simulink library "lib_transmission2"  (Simulink 10.1)
settings: Solver=VariableStepAuto  StartTime=0.0  StopTime=10.0  RelTol=1e-3
undefined symbols (not defined in the file or in its folder): cyc_mph, fc_map_spd, fc_max_trq, fc_spd_scale, fc_trq_scale, fd_inertia, fd_loss, fd_ratio, gb_gear_number_lookup, gb_gears_num, gb_inertia, gb_loss_const, gb_loss_input_spd_coeff, gb_loss_input_trq_coeff, gb_loss_output_spd_coeff, gb_loss_output_trq_coeff, gb_num_init, gb_ratio, gb_shift_delay, gb_spd_scale, gb_trq_scale, htc_inertia, htc_k_adv, htc_k_adv_coast, htc_lockup, htc_lockup_load, htc_lockup_spd, htc_lu_gear_range, htc_max_coast_tr, htc_min_coast_tr, htc_pump_loss_spd, htc_pump_loss_trq_lockup, htc_pump_loss_trq_unlock, htc_sr, htc_sr_coast, htc_tr, htc_tr_coast, htc_unlock_spd, mc_map_spd, mc_max_trq, mc_overtrq_factor, mc_spd_scale, mc_trq_scale, tc_loss, tc_mc_to_fc_ratio, tx_eff_map, tx_map_spd, tx_map_trq, tx_pg_r, tx_pg_s, tx_speed_dep, vc_clutch_bool, vc_idle_spd, vc_launch_spd, wh_radius
undefined symbols (not defined in the file): gb_dnshift_load, gb_dnshift_spd, gb_map_spd_out, gb_map_trq_in, gb_map_trq_out, gb_upshift_load, gb_upshift_spd, logFlag
libraries: lib_controls x1, lib_etc x1, lib_controls2 x1, lib_transmission x1
(part 12 of 17)

== system lib_transmission2/Gearbox Control/automatic transmission gearbox and htc advanced lock-up logic for htc shift logic for gearbox/gearbox control for use w/ AT/Speed Dependent Shifting ==
  note: storing shifting and gear ratio
      | information to workspace
  note: decel case
  note: accel case
  note: accel
      | case
  note: decel
      | case
  note: delta speed
  note: SPEED
      | DEPENDENT
      | SHIFT
      | SIGNAL
  "velocity required (limited) " : Inport
  Look-Up Table (gear for downshift) : Lookup  InputValues="tx_spd_dep_dnshift(:,1)   % vector of speeds m/s"  Table="tx_spd_dep_dnshift(:,2)  % gear number--must be step function"  SaturateOnIntegerOverflow=on
  Look-Up Table (gear for upshift) : Lookup  InputValues="tx_spd_dep_upshift(:,1)   % vector of speeds in m/s"  Table="tx_spd_dep_upshift(:,2)  % gear number--must be step function"  SaturateOnIntegerOverflow=on
  Mux : Mux  Inputs=2
  Mux2 : Mux  Inputs=2
  New gear ratio : ToWorkspace  VariableName=new_gear_ratio
      settings: MaxDataPoints=50000
  Rounding Function : Rounding  Operator=round
  Rounding Function1 : Rounding  Operator=round
  Saturation4 : Saturate  UpperLimit=gb_gears_num  LowerLimit=1
  Saturation5 : Saturate  UpperLimit=gb_gears_num  LowerLimit=1
  "delta speed (\"+\" is acceleration)" : Sum  Inputs=-+  SaturateOnIntegerOverflow=on
  gear ratio6 : Lookup  InputValues=[1:length(gb_ratio)]  Table=gb_ratio  SaturateOnIntegerOverflow=on
  gear ratio8 : Lookup  InputValues=[1:length(gb_ratio)]  Table=gb_ratio  SaturateOnIntegerOverflow=on
  prev veh speed : Memory  InitialCondition=1
  shifting : Subsystem  AncestorBlock=lib_controls/SubSystem/shifting
  shifting1 : Subsystem  AncestorBlock=lib_controls/SubSystem/shifting
  switch for gear number : Switch  Threshold=eps  SaturateOnIntegerOverflow=on  InputSameDT=on
  switch for gear ratio and shifting (muxed) : Switch  Threshold=eps  SaturateOnIntegerOverflow=on  InputSameDT=on
  total fuel used (gal) : ToWorkspace  VariableName=neg_gear_num
      settings: MaxDataPoints=50000
  gear ratio and shifting : Outport
  gear number : Outport  Port=2
  wires:
  Rounding Function1/1 -> Saturation5/1
  Look-Up Table (gear for downshift)/1 -> Rounding Function1/1
  Rounding Function/1 -> Saturation4/1
  Look-Up Table (gear for upshift)/1 -> Rounding Function/1
  "delta speed (\"+\" is acceleration)"/1 -> switch for gear ratio and shifting (muxed)/2, switch for gear number/2
  switch for gear number/1 -> gear number/1
  switch for gear ratio and shifting (muxed)/1 -> gear ratio and shifting/1, New gear ratio/1
  Saturation4/1 -> gear ratio6/1, shifting1/1(gear number), switch for gear number/1
  shifting1/1(out_1) -> Mux/2
  gear ratio6/1 -> Mux/1
  Saturation5/1 -> shifting/1(gear number), gear ratio8/1, total fuel used (gal)/1, switch for gear number/3
  gear ratio8/1 -> Mux2/1
  shifting/1(out_1) -> Mux2/2
  Mux/1 -> switch for gear ratio and shifting (muxed)/1
  Mux2/1 -> switch for gear ratio and shifting (muxed)/3
  prev veh speed/1 -> "delta speed (\"+\" is acceleration)"/1
  "velocity required (limited) "/1 -> Look-Up Table (gear for upshift)/1, Look-Up Table (gear for downshift)/1, "delta speed (\"+\" is acceleration)"/2, prev veh speed/1

== system lib_transmission2/Gearbox Control/automatic transmission gearbox and htc advanced lock-up logic for htc shift logic for gearbox/gearbox control for use w/ AT/allow downshift? ==
  prev gearnum : Inport
  Logical Operator : Logic  Operator=NOR
  Memory : Memory  InitialCondition=1
  Memory1 : Memory  InitialCondition=1
  Relational Operator1 : RelationalOperator  Operator=>  RndMeth=Nearest  InputSameDT=on
  Relational Operator2 : RelationalOperator  Operator=>  RndMeth=Nearest  InputSameDT=on
  allow shift : Outport  InitialOutput=0
  wires:
  Logical Operator/1 -> allow shift/1
  prev gearnum/1 -> Relational Operator1/1, Memory/1, Relational Operator2/1
  Relational Operator1/1 -> Logical Operator/1
  Memory/1 -> Relational Operator1/2, Memory1/1
  Memory1/1 -> Relational Operator2/2
  Relational Operator2/1 -> Logical Operator/2

== system lib_transmission2/Gearbox Control/automatic transmission gearbox and htc advanced lock-up logic for htc shift logic for gearbox/gearbox control for use w/ AT/downshift  command ==
  prev gear number : Inport
  engine load : Inport  Port=2
  engine speed : Inport  Port=3
  Mux : Mux  Inputs=2
  Relational Operator : RelationalOperator  Operator=>  RndMeth=Nearest  InputSameDT=on
  load fraction : Subsystem  mask(Gear Selector){spd=gb_dnshift_spd, load=gb_dnshift_load}
      mask prompts: spd "Speeds:"; load "Load Fractions:"
      mask help:
      | This block will perform a linear interplation (extrapolation outside of bounds) to determine the shift point load fraction associated with the current gear number and speed.
      |
      | The Speeds parameter should be defined as an array of vectors containing speeds for each gear number.  The Load Fractions parameter should be defined as a array of vectors containing load fractions indexed by the speeds in the Speeds parameter for each gear number.
      mask Help:
      | Reference the base workspace variables - gb_**shift_spd and gb_**shift_load  where ** is either up for upshift conditions or dn for downshift conditions.
      | 
      | Or define the arrays as follows:
      | 
      | {[spd1 spd2 spd3 spd4]; [spd1 spd2 spd3 spd4]; ...}
      | 
      | {[load1 load2 load3 load4]; [load1 load2 load3 load4]; ...}
      | 
      | where each array contains one row for each gear in the gearbox.  Speeds should be defined in rad/s and loads as a decimal fraction.
  command : Outport  InitialOutput=0
  wires:
  Relational Operator/1 -> command/1
  engine speed/1 -> Mux/2
  prev gear number/1 -> Mux/1
  engine load/1 -> Relational Operator/1
  Mux/1 -> load fraction/1(In1)
  load fraction/1(Out1) -> Relational Operator/2

== system lib_transmission2/Gearbox Control/automatic transmission gearbox and htc advanced lock-up logic for htc shift logic for gearbox/gearbox control for use w/ AT/downshift  command1 ==
  prev gear number : Inport
  engine load : Inport  Port=2
  engine speed : Inport  Port=3
  Mux : Mux  Inputs=2
  Relational Operator : RelationalOperator  Operator=>  RndMeth=Nearest  InputSameDT=on
  load fraction : Subsystem  mask(Gear Selector){spd=gb_dnshift_spd, load=gb_dnshift_load}
      mask prompts: spd "Speeds:"; load "Load Fractions:"
      mask help:
      | This block will perform a linear interplation (extrapolation outside of bounds) to determine the shift point load fraction associated with the current gear number and speed.
      |
      | The Speeds parameter should be defined as an array of vectors containing speeds for each gear number.  The Load Fractions parameter should be defined as a array of vectors containing load fractions indexed by the speeds in the Speeds parameter for each gear number.
      mask Help:
      | Reference the base workspace variables - gb_**shift_spd and gb_**shift_load  where ** is either up for upshift conditions or dn for downshift conditions.
      | 
      | Or define the arrays as follows:
      | 
      | {[spd1 spd2 spd3 spd4]; [spd1 spd2 spd3 spd4]; ...}
      | 
      | {[load1 load2 load3 load4]; [load1 load2 load3 load4]; ...}
      | 
      | where each array contains one row for each gear in the gearbox.  Speeds should be defined in rad/s and loads as a decimal fraction.
  command : Outport  InitialOutput=0
  wires:
  engine speed/1 -> Mux/2
  load fraction/1(Out1) -> Relational Operator/2
  Mux/1 -> load fraction/1(In1)
  engine load/1 -> Relational Operator/1
  prev gear number/1 -> Mux/1
  Relational Operator/1 -> command/1

== system lib_transmission2/Gearbox Control/automatic transmission gearbox and htc advanced lock-up logic for htc shift logic for gearbox/gearbox control for use w/ AT/est. engine trq and spd ==
  prev gear number : Inport
  " prev eta_gb" : Inport  Port=2
  gb_trq_out_r : Inport  Port=3
  gb_spd_out_r : Inport  Port=4
  Block NOTES : Subsystem
      mask Display: disp('Block\nNOTES')
  Constant2 : Constant  Value=[1 1]
  Constant5 : Constant  Value=0
  Demux : Demux  Outputs=2
  K_adv : Subsystem
  Logical Operator : Logic
  Logical Operator1 : Logic  Operator=NOT  Inputs=1
  Memory : Memory
  Mux1 : Mux  Inputs=2
  Mux2 : Mux  Inputs=2
  Relational Operator1 : RelationalOperator  Operator=>  RndMeth=Nearest  InputSameDT=on
  SR Look-Up Table SR=wout/win : Lookup  InputValues=htc_k_adv  Table=htc_sr  SaturateOnIntegerOverflow=on
  Saturation1 : Saturate  UpperLimit=1  LowerLimit=0.7
  Saturation2 : Saturate  UpperLimit=inf  LowerLimit=0
  Switch : Switch  Threshold=eps  SaturateOnIntegerOverflow=on  InputSameDT=on
  TR Look-Up Table TR=Tout/Tin : Lookup  InputValues=htc_k_adv  Table=htc_tr  SaturateOnIntegerOverflow=on
  TR,SR : Mux  Inputs=2
  est eng trq : Sum  SaturateOnIntegerOverflow=on
  gear ratio1 : Lookup  InputValues=[1:length(gb_ratio)]  Table=gb_ratio  SaturateOnIntegerOverflow=on
  ~eng trq and spd : Product  Inputs=*/  SaturateOnIntegerOverflow=on
  ~gb_spd_in_r : Product  SaturateOnIntegerOverflow=on
  ~gb_trq_in_r : Product  Inputs=//*  SaturateOnIntegerOverflow=on
  est eng trq (Nm) : Outport
  est eng spd (rad/s) : Outport  Port=2
  gb_spd_in_est (rad/s)1 : Outport  Port=3
  wires:
  est eng trq/1 -> Mux1/1, Relational Operator1/1, Mux2/1
  ~gb_trq_in_r/1 -> est eng trq/1
  ~gb_spd_in_r/1 -> Mux2/2, gb_spd_in_est (rad/s)1/1, Mux1/2
  [acc_mech_trq_est] -> est eng trq/2
  SR Look-Up Table SR=wout/win/1 -> TR,SR/2
  TR Look-Up Table TR=Tout/Tin/1 -> TR,SR/1
  K_adv/1(K_adv) -> SR Look-Up Table SR=wout/win/1, TR Look-Up Table TR=Tout/Tin/1
  Mux2/1 -> K_adv/1("Req'd output trq and spd (Nm), (rad/s)")
  ~eng trq and spd/1 -> Demux/1
  Mux1/1 -> ~eng trq and spd/1
  [locked_up] -> Memory/1
  Logical Operator/1 -> Switch/2
  Logical Operator1/1 -> Logical Operator/2
  Memory/1 -> Logical Operator1/1
  Demux/1 -> est eng trq (Nm)/1
  prev gear number/1 -> gear ratio1/1
  Relational Operator1/1 -> Logical Operator/1
  Constant5/1 -> Relational Operator1/2
  Saturation2/1 -> est eng spd (rad/s)/1
  Demux/2 -> Saturation2/1
  Saturation1/1 -> ~gb_trq_in_r/2
  " prev eta_gb"/1 -> Saturation1/1
  Switch/1 -> ~eng trq and spd/2
  Constant2/1 -> Switch/3
  TR,SR/1 -> Switch/1
  gear ratio1/1 -> ~gb_spd_in_r/1, ~gb_trq_in_r/1
  gb_spd_out_r/1 -> ~gb_spd_in_r/2
  gb_trq_out_r/1 -> ~gb_trq_in_r/3

== system lib_transmission2/Gearbox Control/automatic transmission gearbox and htc advanced lock-up logic for htc shift logic for gearbox/gearbox control for use w/ AT/est. engine trq and spd assuming lockup ==
  new gear number : Inport
  " prev eta_gb" : Inport  Port=2
  gb_trq_out_r : Inport  Port=3
  gb_spd_in_est : Inport  Port=4
  Block NOTES : Subsystem
      mask Display: disp('Block\nNOTES')
  Memory : Memory  InitialCondition=gb_ratio(1)
  Saturation1 : Saturate  UpperLimit=1  LowerLimit=0.7
  Saturation2 : Saturate  UpperLimit=inf  LowerLimit=0
  est eng trq : Sum  SaturateOnIntegerOverflow=on
  gear ratio1 : Lookup  InputValues=[1:length(gb_ratio)]  Table=gb_ratio  SaturateOnIntegerOverflow=on
  ~gb_spd_in_r : Product  Inputs=*/*  SaturateOnIntegerOverflow=on
  ~gb_trq_in_r : Product  Inputs=//*  SaturateOnIntegerOverflow=on
  est eng trq (Nm) : Outport
  est eng spd (rad/s) : Outport  Port=2
  wires:
  ~gb_spd_in_r/1 -> Saturation2/1
  est eng trq/1 -> est eng trq (Nm)/1
  ~gb_trq_in_r/1 -> est eng trq/1
  [acc_mech_trq_est] -> est eng trq/2
  gb_spd_in_est/1 -> ~gb_spd_in_r/3
  Memory/1 -> ~gb_spd_in_r/2
  Saturation2/1 -> est eng spd (rad/s)/1
  new gear number/1 -> gear ratio1/1
  gb_trq_out_r/1 -> ~gb_trq_in_r/3
  gear ratio1/1 -> Memory/1, ~gb_spd_in_r/1, ~gb_trq_in_r/1
  " prev eta_gb"/1 -> Saturation1/1
  Saturation1/1 -> ~gb_trq_in_r/2

== system lib_transmission2/Gearbox Control/automatic transmission gearbox and htc advanced lock-up logic for htc shift logic for gearbox/gearbox control for use w/ AT/htc lockup logic ==
  engine load (%) : Inport
  gear num : Inport  Port=2
  Constant1 : Constant  Value=0.5
  Constant2 : Constant  Value=0
  Constant3 : Constant  Value=0
  Constant4 : Constant  Value=-1
  Logical Operator : Logic  Operator=NOR
  Memory1 : Memory  InitialCondition=1
  Memory2 : Memory  InitialCondition=1
  Memory3 : Memory  InitialCondition=1
  Relational Operator : RelationalOperator  RndMeth=Nearest  InputSameDT=on
  Relational Operator1 : RelationalOperator  Operator=>  RndMeth=Nearest  InputSameDT=on
  Relational Operator2 : RelationalOperator  Operator=<  RndMeth=Nearest  InputSameDT=on
  Relational Operator3 : RelationalOperator  Operator=<  RndMeth=Nearest  InputSameDT=on
  Saturation1 : Saturate  UpperLimit=1  LowerLimit=0
  Switch{,1..3} (4 alike) : Switch  Threshold=0.5  SaturateOnIntegerOverflow=on  InputSameDT=on
  current lock/unlock  status : Sum  SaturateOnIntegerOverflow=on
  lock-up in high gears : Lookup  InputValues=[1:length(htc_lockup)]  Table=htc_lockup  SaturateOnIntegerOverflow=on
  lock-up in this gear : Lookup  InputValues=htc_lockup_load  Table=htc_lockup_spd  SaturateOnIntegerOverflow=on
  lock/unlock  gear range : Lookup  InputValues=[1:length(htc_lockup)]  Table=htc_lu_gear_range  SaturateOnIntegerOverflow=on
  unlock in this gear : Lookup  InputValues=htc_lockup_load  Table=htc_unlock_spd  SaturateOnIntegerOverflow=on
  htc L/UL : Outport
  wires:
  Constant1/1 -> Relational Operator/2, Relational Operator1/1
  gear num/1 -> lock-up in high gears/1, lock/unlock  gear range/1
  lock-up in high gears/1 -> Relational Operator/1
  Relational Operator/1 -> Switch/2, Switch/1
  Switch/1 -> htc L/UL/1, Memory1/1
  lock/unlock  gear range/1 -> Relational Operator1/2
  lock-up in this gear/1 -> Relational Operator2/1
  unlock in this gear/1 -> Relational Operator3/2
  Relational Operator1/1 -> Switch1/2
  Constant2/1 -> Switch1/1
  Switch1/1 -> Switch/3
  Saturation1/1 -> Switch1/3
  Relational Operator2/1 -> Logical Operator/1, Switch3/2, Switch3/1
  Relational Operator3/1 -> Logical Operator/2
  Logical Operator/1 -> Switch2/2
  Constant3/1 -> Switch2/3
  Switch3/1 -> Switch2/1
  Constant4/1 -> Switch3/3
  current lock/unlock  status/1 -> Saturation1/1
  Memory1/1 -> current lock/unlock  status/1
  Switch2/1 -> current lock/unlock  status/2
  Memory2/1 -> Relational Operator2/2, Relational Operator3/1
  Memory3/1 -> lock-up in this gear/1, unlock in this gear/1
  engine load (%)/1 -> Memory3/1
  [gb_trq_out_a] -> Memory2/1

== system lib_transmission2/Gearbox Control/automatic transmission gearbox and htc advanced lock-up logic for htc shift logic for gearbox/gearbox control for use w/ AT/shifting1 ==
  gear number : Inport
  Constant : Constant  Value=gb_shift_delay-1e-6
  Relational Operator : RelationalOperator  Operator=<  RndMeth=Nearest  InputSameDT=on
  time since last shift : Subsystem
      mask Display: disp('time since\nlast shift')
  out_1 : Outport  InitialOutput=0
  wires:
  Relational Operator/1 -> out_1/1
  gear number/1 -> time since last shift/1(in_1)
  Constant/1 -> Relational Operator/2
  time since last shift/1(out_1) -> Relational Operator/1

== system lib_transmission2/Gearbox Control/automatic transmission gearbox and htc advanced lock-up logic for htc shift logic for gearbox/gearbox control for use w/ AT/upshift  command ==
  prev gear number : Inport
  engine load : Inport  Port=2
  engine speed : Inport  Port=3
  Mux : Mux  Inputs=2
  Relational Operator : RelationalOperator  Operator=<  RndMeth=Nearest  InputSameDT=on
  load fraction : Subsystem  mask(Gear Selector){spd=gb_upshift_spd, load=gb_upshift_load}
      mask prompts: spd "Speeds:"; load "Load Fractions:"
      mask help:
      | This block will perform a linear interplation (extrapolation outside of bounds) to determine the shift point load fraction associated with the current gear number and speed.
      |
      | The Speeds parameter should be defined as an array of vectors containing speeds for each gear number.  The Load Fractions parameter should be defined as a array of vectors containing load fractions indexed by the speeds in the Speeds parameter for each gear number.
      mask Help:
      | Reference the base workspace variables - gb_**shift_spd and gb_**shift_load  where ** is either up for upshift conditions or dn for downshift conditions.
      | 
      | Or define the arrays as follows:
      | 
      | {[spd1 spd2 spd3 spd4]; [spd1 spd2 spd3 spd4]; ...}
      | 
      | {[load1 load2 load3 load4]; [load1 load2 load3 load4]; ...}
      | 
      | where each array contains one row for each gear in the gearbox.  Speeds should be defined in rad/s and loads as a decimal fraction.
  command : Outport  InitialOutput=0
  wires:
  Relational Operator/1 -> command/1
  engine speed/1 -> Mux/2
  Mux/1 -> load fraction/1(In1)
  prev gear number/1 -> Mux/1
  engine load/1 -> Relational Operator/1
  load fraction/1(Out1) -> Relational Operator/2

== system lib_transmission2/Gearbox Control/automatic transmission gearbox and htc standard lockup logic for htc shift logic for gearbox/gearbox control for use w/ AT/Block NOTES ==
  note: This gearbox control block computes the current gear number given the gearbox's
      | req'd output torque and speed and an estimate its efficiency.  Upshifts occur, given a
      | certain engine speed,  when the estimated engine load falls below the upshift curve
      | in engine speed/load space, and downshifts likewise occur when estimated engine
      | load rises above the downshift curve.  Separate upshift and downshift curves are
      | defined for each gear.  An upshift may not be immediately followed by a downshift.
      | If the tires are about to slip, don't upshift unless the engine would be at max. speed.
      | Enforce this rule by setting the load to 1 when the tires are about to slip.
  note: Lock-up of the HTC occurs when it is supposed to for the current gear, AND
      | the transmission isn't shifting, AND
      | the lockup wouldn't precipitate an immediate downshift.

== system lib_transmission2/Gearbox Control/automatic transmission gearbox and htc standard lockup logic for htc shift logic for gearbox/gearbox control for use w/ AT/allow downshift? ==
  prev gearnum : Inport
  Logical Operator : Logic  Operator=NOR
  Memory : Memory  InitialCondition=1
  Memory1 : Memory  InitialCondition=1
  Relational Operator1 : RelationalOperator  Operator=>  RndMeth=Nearest  InputSameDT=on
  Relational Operator2 : RelationalOperator  Operator=>  RndMeth=Nearest  InputSameDT=on
  allow shift : Outport  InitialOutput=0
  wires:
  Relational Operator2/1 -> Logical Operator/2
  Memory1/1 -> Relational Operator2/2
  Memory/1 -> Memory1/1, Relational Operator1/2
  Relational Operator1/1 -> Logical Operator/1
  prev gearnum/1 -> Relational Operator2/1, Memory/1, Relational Operator1/1
  Logical Operator/1 -> allow shift/1

== system lib_transmission2/Gearbox Control/automatic transmission gearbox and htc standard lockup logic for htc shift logic for gearbox/gearbox control for use w/ AT/downshift  command ==
  prev gear number : Inport
  engine load : Inport  Port=2
  engine speed : Inport  Port=3
  Mux : Mux  Inputs=2
  Relational Operator : RelationalOperator  Operator=>  RndMeth=Nearest  InputSameDT=on
  load fraction : Subsystem  mask(Gear Selector){spd=gb_dnshift_spd, load=gb_dnshift_load}
      mask prompts: spd "Speeds:"; load "Load Fractions:"
      mask help:
      | This block will perform a linear interplation (extrapolation outside of bounds) to determine the shift point load fraction associated with the current gear number and speed.
      |
      | The Speeds parameter should be defined as an array of vectors containing speeds for each gear number.  The Load Fractions parameter should be defined as a array of vectors containing load fractions indexed by the speeds in the Speeds parameter for each gear number.
      mask Help:
      | Reference the base workspace variables - gb_**shift_spd and gb_**shift_load  where ** is either up for upshift conditions or dn for downshift conditions.
      | 
      | Or define the arrays as follows:
      | 
      | {[spd1 spd2 spd3 spd4]; [spd1 spd2 spd3 spd4]; ...}
      | 
      | {[load1 load2 load3 load4]; [load1 load2 load3 load4]; ...}
      | 
      | where each array contains one row for each gear in the gearbox.  Speeds should be defined in rad/s and loads as a decimal fraction.
  command : Outport  InitialOutput=0
  wires:
  load fraction/1(Out1) -> Relational Operator/2
  Mux/1 -> load fraction/1(In1)
  engine load/1 -> Relational Operator/1
  prev gear number/1 -> Mux/1
  engine speed/1 -> Mux/2
  Relational Operator/1 -> command/1

== system lib_transmission2/Gearbox Control/automatic transmission gearbox and htc standard lockup logic for htc shift logic for gearbox/gearbox control for use w/ AT/downshift  command1 ==
  prev gear number : Inport
  engine load : Inport  Port=2
  engine speed : Inport  Port=3
  Mux : Mux  Inputs=2
  Relational Operator : RelationalOperator  Operator=>  RndMeth=Nearest  InputSameDT=on
  load fraction : Subsystem  mask(Gear Selector){spd=gb_dnshift_spd, load=gb_dnshift_load}
      mask prompts: spd "Speeds:"; load "Load Fractions:"
      mask help:
      | This block will perform a linear interplation (extrapolation outside of bounds) to determine the shift point load fraction associated with the current gear number and speed.
      |
      | The Speeds parameter should be defined as an array of vectors containing speeds for each gear number.  The Load Fractions parameter should be defined as a array of vectors containing load fractions indexed by the speeds in the Speeds parameter for each gear number.
      mask Help:
      | Reference the base workspace variables - gb_**shift_spd and gb_**shift_load  where ** is either up for upshift conditions or dn for downshift conditions.
      | 
      | Or define the arrays as follows:
      | 
      | {[spd1 spd2 spd3 spd4]; [spd1 spd2 spd3 spd4]; ...}
      | 
      | {[load1 load2 load3 load4]; [load1 load2 load3 load4]; ...}
      | 
      | where each array contains one row for each gear in the gearbox.  Speeds should be defined in rad/s and loads as a decimal fraction.
  command : Outport  InitialOutput=0
  wires:
  Relational Operator/1 -> command/1
  prev gear number/1 -> Mux/1
  engine load/1 -> Relational Operator/1
  Mux/1 -> load fraction/1(In1)
  load fraction/1(Out1) -> Relational Operator/2
  engine speed/1 -> Mux/2

== system lib_transmission2/Gearbox Control/automatic transmission gearbox and htc standard lockup logic for htc shift logic for gearbox/gearbox control for use w/ AT/est. engine trq and spd ==
  prev gear number : Inport
  " prev eta_gb" : Inport  Port=2
  gb_trq_out_r : Inport  Port=3
  gb_spd_out_r : Inport  Port=4
  Block NOTES : Subsystem
      mask Display: disp('Block\nNOTES')
  Constant2 : Constant  Value=[1 1]
  Constant5 : Constant  Value=0
  Demux : Demux  Outputs=2
  K_adv : Subsystem
  Logical Operator : Logic
  Logical Operator1 : Logic  Operator=NOT  Inputs=1
  Mux1 : Mux  Inputs=2
  Mux2 : Mux  Inputs=2
  Relational Operator1 : RelationalOperator  Operator=>  RndMeth=Nearest  InputSameDT=on
  SR Look-Up Table SR=wout/win : Lookup  InputValues=htc_k_adv  Table=htc_sr  SaturateOnIntegerOverflow=on
  Saturation1 : Saturate  UpperLimit=1  LowerLimit=0.7
  Saturation2 : Saturate  UpperLimit=inf  LowerLimit=0
  Switch : Switch  Threshold=eps  SaturateOnIntegerOverflow=on  InputSameDT=on
  TR Look-Up Table TR=Tout/Tin : Lookup  InputValues=htc_k_adv  Table=htc_tr  SaturateOnIntegerOverflow=on
  TR,SR : Mux  Inputs=2
  est eng trq : Sum  SaturateOnIntegerOverflow=on
  gear ratio : Lookup  InputValues=[1:length(gb_ratio)]  Table=gb_ratio  SaturateOnIntegerOverflow=on
  ~eng trq and spd : Product  Inputs=*/  SaturateOnIntegerOverflow=on
  ~gb_spd_in_r : Product  SaturateOnIntegerOverflow=on
  ~gb_trq_in_r : Product  Inputs=//*  SaturateOnIntegerOverflow=on
  est eng trq (Nm) : Outport
  est eng spd (rad/s) : Outport  Port=2
  gb_spd_in_est (rad/s) : Outport  Port=3
  wires:
  gb_trq_out_r/1 -> ~gb_trq_in_r/3
  gb_spd_out_r/1 -> ~gb_spd_in_r/2
  gear ratio/1 -> ~gb_trq_in_r/1, ~gb_spd_in_r/1
  TR,SR/1 -> Switch/1
  Constant2/1 -> Switch/3
  Switch/1 -> ~eng trq and spd/2
  " prev eta_gb"/1 -> Saturation1/1
  Saturation1/1 -> ~gb_trq_in_r/2
  Demux/2 -> Saturation2/1
  Saturation2/1 -> est eng spd (rad/s)/1
  Constant5/1 -> Relational Operator1/2
  Relational Operator1/1 -> Logical Operator/1
  prev gear number/1 -> gear ratio/1
  Demux/1 -> est eng trq (Nm)/1
  Logical Operator1/1 -> Logical Operator/2
  Logical Operator/1 -> Switch/2
  [locked_up_last] -> Logical Operator1/1
  Mux1/1 -> ~eng trq and spd/1
  ~eng trq and spd/1 -> Demux/1
  Mux2/1 -> K_adv/1("Req'd output trq and spd (Nm), (rad/s)")
  K_adv/1(K_adv) -> TR Look-Up Table TR=Tout/Tin/1, SR Look-Up Table SR=wout/win/1
  TR Look-Up Table TR=Tout/Tin/1 -> TR,SR/1
  SR Look-Up Table SR=wout/win/1 -> TR,SR/2
  [acc_mech_trq_est] -> est eng trq/2
  ~gb_spd_in_r/1 -> Mux1/2, gb_spd_in_est (rad/s)/1, Mux2/2
  ~gb_trq_in_r/1 -> est eng trq/1
  est eng trq/1 -> Mux2/1, Relational Operator1/1, Mux1/1

== system lib_transmission2/Gearbox Control/automatic transmission gearbox and htc standard lockup logic for htc shift logic for gearbox/gearbox control for use w/ AT/est. engine trq and spd assuming lockup ==
  new gear number : Inport
  " prev eta_gb" : Inport  Port=2
  gb_trq_out_r : Inport  Port=3
  gb_spd_in_est : Inport  Port=4
  Block NOTES : Subsystem
      mask Display: disp('Block\nNOTES')
  Memory : Memory  InitialCondition=gb_ratio(1)
  Saturation1 : Saturate  UpperLimit=1  LowerLimit=0.7
  Saturation2 : Saturate  UpperLimit=inf  LowerLimit=0
  est eng trq : Sum  SaturateOnIntegerOverflow=on
  gear ratio1 : Lookup  InputValues=[1:length(gb_ratio)]  Table=gb_ratio  SaturateOnIntegerOverflow=on
  ~gb_spd_in_r : Product  Inputs=*/*  SaturateOnIntegerOverflow=on
  ~gb_trq_in_r : Product  Inputs=//*  SaturateOnIntegerOverflow=on
  est eng trq (Nm) : Outport
  est eng spd (rad/s) : Outport  Port=2
  wires:
  Saturation1/1 -> ~gb_trq_in_r/2
  " prev eta_gb"/1 -> Saturation1/1
  gear ratio1/1 -> ~gb_trq_in_r/1, ~gb_spd_in_r/1, Memory/1
  gb_trq_out_r/1 -> ~gb_trq_in_r/3
  new gear number/1 -> gear ratio1/1
  Saturation2/1 -> est eng spd (rad/s)/1
  Memory/1 -> ~gb_spd_in_r/2
  gb_spd_in_est/1 -> ~gb_spd_in_r/3
  [acc_mech_trq_est] -> est eng trq/2
  ~gb_trq_in_r/1 -> est eng trq/1
  est eng trq/1 -> est eng trq (Nm)/1
  ~gb_spd_in_r/1 -> Saturation2/1

== system lib_transmission2/Gearbox Control/automatic transmission gearbox and htc standard lockup logic for htc shift logic for gearbox/gearbox control for use w/ AT/shifting1 ==
  gear number : Inport
  Constant : Constant  Value=gb_shift_delay-1e-6
  Relational Operator : RelationalOperator  Operator=<  RndMeth=Nearest  InputSameDT=on
  time since last shift : Subsystem
      mask Display: disp('time since\nlast shift')
  out_1 : Outport  InitialOutput=0
  wires:
  time since last shift/1(out_1) -> Relational Operator/1
  Constant/1 -> Relational Operator/2
  gear number/1 -> time since last shift/1(in_1)
  Relational Operator/1 -> out_1/1

== system lib_transmission2/Gearbox Control/automatic transmission gearbox and htc standard lockup logic for htc shift logic for gearbox/gearbox control for use w/ AT/upshift  command ==
  prev gear number : Inport
  engine load : Inport  Port=2
  engine speed : Inport  Port=3
  Mux : Mux  Inputs=2
  Relational Operator : RelationalOperator  Operator=<  RndMeth=Nearest  InputSameDT=on
  load fraction : Subsystem  mask(Gear Selector){spd=gb_upshift_spd, load=gb_upshift_load}
      mask prompts: spd "Speeds:"; load "Load Fractions:"
      mask help:
      | This block will perform a linear interplation (extrapolation outside of bounds) to determine the shift point load fraction associated with the current gear number and speed.
      |
      | The Speeds parameter should be defined as an array of vectors containing speeds for each gear number.  The Load Fractions parameter should be defined as a array of vectors containing load fractions indexed by the speeds in the Speeds parameter for each gear number.
      mask Help:
      | Reference the base workspace variables - gb_**shift_spd and gb_**shift_load  where ** is either up for upshift conditions or dn for downshift conditions.
      | 
      | Or define the arrays as follows:
      | 
      | {[spd1 spd2 spd3 spd4]; [spd1 spd2 spd3 spd4]; ...}
      | 
      | {[load1 load2 load3 load4]; [load1 load2 load3 load4]; ...}
      | 
      | where each array contains one row for each gear in the gearbox.  Speeds should be defined in rad/s and loads as a decimal fraction.
  command : Outport  InitialOutput=0
  wires:
  load fraction/1(Out1) -> Relational Operator/2
  engine load/1 -> Relational Operator/1
  prev gear number/1 -> Mux/1
  Mux/1 -> load fraction/1(In1)
  engine speed/1 -> Mux/2
  Relational Operator/1 -> command/1

== system lib_transmission2/Gearbox Control/time lookup shift logic for gearbox/lookup/shifting determination ==
  gear number : Inport
  Constant : Constant  Value=gb_shift_delay-1e-6
  Relational Operator : RelationalOperator  Operator=<  RndMeth=Nearest  InputSameDT=on
  time since last shift : Subsystem
      mask Display: disp('time since\nlast shift')
  out_1 : Outport  InitialOutput=0
  wires:
  time since last shift/1(out_1) -> Relational Operator/1
  Constant/1 -> Relational Operator/2
  gear number/1 -> time since last shift/1(in_1)
  Relational Operator/1 -> out_1/1

== system lib_transmission2/Gearbox Control/vehicle speed dependent shift logic for gearbox/speed dependent/Speed Dependent Shifting ==
  note: storing shifting and gear ratio
      | information to workspace
  note: decel case
  note: accel case
  note: accel
      | case
  note: decel
      | case
  note: delta speed
  note: SPEED
      | DEPENDENT
      | SHIFT
      | SIGNAL
  "velocity required (limited) " : Inport
  Look-Up Table (gear for downshift) : Lookup  InputValues="tx_spd_dep_dnshift(:,1)   % vector of speeds m/s"  Table="tx_spd_dep_dnshift(:,2)  % gear number--must be step function"  SaturateOnIntegerOverflow=on
  Look-Up Table (gear for upshift) : Lookup  InputValues="tx_spd_dep_upshift(:,1)   % vector of speeds in m/s"  Table="tx_spd_dep_upshift(:,2)  % gear number--must be step function"  SaturateOnIntegerOverflow=on
  Mux : Mux  Inputs=2
  Mux2 : Mux  Inputs=2
  New gear ratio : ToWorkspace  VariableName=new_gear_ratio
      settings: MaxDataPoints=50000
  Rounding Function : Rounding  Operator=round
  Rounding Function1 : Rounding  Operator=round
  Saturation4 : Saturate  UpperLimit=gb_gears_num  LowerLimit=1
  Saturation5 : Saturate  UpperLimit=gb_gears_num  LowerLimit=1
  "delta speed (\"+\" is acceleration)" : Sum  Inputs=-+  SaturateOnIntegerOverflow=on
  gear ratio6 : Lookup  InputValues=[1:length(gb_ratio)]  Table=gb_ratio  SaturateOnIntegerOverflow=on
  gear ratio8 : Lookup  InputValues=[1:length(gb_ratio)]  Table=gb_ratio  SaturateOnIntegerOverflow=on
  prev veh speed : Memory  InitialCondition=1
  shifting : Subsystem
  shifting1 : Subsystem
  switch for gear number : Switch  Threshold=eps  SaturateOnIntegerOverflow=on  InputSameDT=on
  switch for gear ratio and shifting (muxed) : Switch  Threshold=eps  SaturateOnIntegerOverflow=on  InputSameDT=on
  total fuel used (gal) : ToWorkspace  VariableName=neg_gear_num
      settings: MaxDataPoints=50000
  gear ratio and shifting : Outport
  gear number : Outport  Port=2
  wires:
  Rounding Function1/1 -> Saturation5/1
  Look-Up Table (gear for downshift)/1 -> Rounding Function1/1
  Rounding Function/1 -> Saturation4/1
  Look-Up Table (gear for upshift)/1 -> Rounding Function/1
  "delta speed (\"+\" is acceleration)"/1 -> switch for gear ratio and shifting (muxed)/2, switch for gear number/2
  switch for gear number/1 -> gear number/1
  switch for gear ratio and shifting (muxed)/1 -> gear ratio and shifting/1, New gear ratio/1
  Saturation4/1 -> gear ratio6/1, shifting1/1(gear number), switch for gear number/1
  shifting1/1(out_1) -> Mux/2
  gear ratio6/1 -> Mux/1
  Saturation5/1 -> shifting/1(gear number), gear ratio8/1, total fuel used (gal)/1, switch for gear number/3
  gear ratio8/1 -> Mux2/1
  shifting/1(out_1) -> Mux2/2
  Mux/1 -> switch for gear ratio and shifting (muxed)/1
  Mux2/1 -> switch for gear ratio and shifting (muxed)/3
  prev veh speed/1 -> "delta speed (\"+\" is acceleration)"/1
  "velocity required (limited) "/1 -> Look-Up Table (gear for upshift)/1, Look-Up Table (gear for downshift)/1, "delta speed (\"+\" is acceleration)"/2, prev veh speed/1

== system lib_transmission2/clutch <cl>/clutch model and interface/clutch model/Adjust for Possible Launch Speed Request ==
  note: If the clutch is disengaged, under certain
      | circumstances, we will want to request that
      | the input speed to the clutch be ramped up to a
      | given launch speed (decided by the controller)
      | so that the clutch can subsequently slip and
      | engage with a more realistic speed matching
  Input Speed Request : Inport
  Constant6 : Constant
  Logical Operator : Logic
  Switch4 : Switch  Threshold=0.5  SaturateOnIntegerOverflow=on  InputSameDT=on
  clutch disengaged : RelationalOperator  Operator===  RndMeth=Nearest  InputSameDT=on
  Input Speed Request Adjusted for Launch Speed : Outport
  wires:
  [launch_speed] -> Switch4/1
  Switch4/1 -> Input Speed Request Adjusted for Launch Speed/1
  Input Speed Request/1 -> Switch4/3
  [clutch_state] -> clutch disengaged/1
  Constant6/1 -> clutch disengaged/2
  [launch_flag] -> Logical Operator/1
  clutch disengaged/1 -> Logical Operator/2
  Logical Operator/1 -> Switch4/2

== system lib_transmission2/clutch <cl>/clutch model and interface/clutch model/enhancedToWorkspace ==
  In1 : Inport
  Terminator : Terminator
  wires:
  In1/1 -> Terminator/1

== system lib_transmission2/clutch <cl>/clutch model and interface/clutch model/enhancedToWorkspace1 ==
  In1 : Inport
  Terminator : Terminator
  wires:
  In1/1 -> Terminator/1

== system lib_transmission2/clutch <cl>/clutch model and interface/clutch model/enhancedToWorkspace2 ==
  In1 : Inport
  Terminator : Terminator
  wires:
  In1/1 -> Terminator/1

== system lib_transmission2/clutch <cl>/clutch model and interface/clutch model/enhancedToWorkspace3 ==
  In1 : Inport
  Terminator : Terminator
  wires:
  In1/1 -> Terminator/1

== system lib_transmission2/clutch <cl>/clutch model and interface/clutch model/enhancedToWorkspace4 ==
  In1 : Inport
  Terminator : Terminator
  wires:
  In1/1 -> Terminator/1

== system lib_transmission2/clutch <cl>/clutch model and interface/clutch model/enhancedToWorkspace5 ==
  In1 : Inport
  Terminator : Terminator
  wires:
  In1/1 -> Terminator/1

== system lib_transmission2/clutch <cl>/clutch model and interface/clutch model/enhancedToWorkspace6 ==
  In1 : Inport
  Terminator : Terminator
  wires:
  In1/1 -> Terminator/1

== system lib_transmission2/clutch <cl>/clutch model and interface/clutch model/enhancedToWorkspace7 ==
  In1 : Inport
  Terminator : Terminator
  wires:
  In1/1 -> Terminator/1

== system lib_transmission2/clutch <cl>/clutch model and interface/clutch model/enhancedToWorkspace8 ==
  In1 : Inport
  Terminator : Terminator
  wires:
  In1/1 -> Terminator/1

== system lib_transmission2/clutch <cl>/clutch model and interface/clutch model/enhancedToWorkspace9 ==
  In1 : Inport
  Terminator : Terminator
  wires:
  In1/1 -> Terminator/1

== system lib_transmission2/clutch <cl>/clutch model and interface/clutch model/help ==

== system lib_transmission2/final drive <fd>/model&interface/model/Block NOTES ==
  note: This final drive model includes loss data, rotational inertia, and a gear reduction.
  note: The loss torque is zero when the gears are not turning,
      | and is applied at the input side of the gear reduction.
  note: The inertia torque is the input torque required to accelerate the
      | final drive's inertia as measured on the input side.

== system lib_transmission2/final drive <fd>/model&interface/model/effect of inertia (Nm) ==
  note: The inertia torque is the input torque required to accelerate the
      | final drive's inertia as measured on the input side.
  fd input speed (rad/s) : Inport
  Gain : Gain  Gain=fd_inertia  SaturateOnIntegerOverflow=on
  d/dt : Derivative
  drag torque (Nm) : Outport  InitialOutput=0
  wires:
  Gain/1 -> drag torque (Nm)/1
  d/dt/1 -> Gain/1
  fd input speed (rad/s)/1 -> d/dt/1

== system lib_transmission2/final drive <fd>/model&interface/model/enhancedToWorkspace ==
  In1 : Inport
  To Workspace : ToWorkspace  VariableName=fd_trq_in_a  SampleTime=-1
  wires:
  In1/1 -> To Workspace/1

== system lib_transmission2/final drive <fd>/model&interface/model/enhancedToWorkspace1 ==
  In1 : Inport
  To Workspace : ToWorkspace  VariableName=fd_spd_in_a  SampleTime=-1
  wires:
  In1/1 -> To Workspace/1

== system lib_transmission2/final drive <fd>/model&interface/model/enhancedToWorkspace2 ==
  In1 : Inport
  To Workspace : ToWorkspace  VariableName=fd_spd_out_a  SampleTime=-1
  wires:
  In1/1 -> To Workspace/1

== system lib_transmission2/final drive <fd>/model&interface/model/enhancedToWorkspace3 ==
  In1 : Inport
  To Workspace : ToWorkspace  VariableName=fd_trq_out_a  SampleTime=-1
  wires:
  In1/1 -> To Workspace/1

== system lib_transmission2/final drive <fd>/model&interface/model/enhancedToWorkspace4 ==
  In1 : Inport
  To Workspace : ToWorkspace  VariableName=fd_spd_in_r  SampleTime=-1
  wires:
  In1/1 -> To Workspace/1

== system lib_transmission2/final drive <fd>/model&interface/model/enhancedToWorkspace5 ==
  In1 : Inport
  To Workspace : ToWorkspace  VariableName=fd_trq_in_r  SampleTime=-1
  wires:
  In1/1 -> To Workspace/1

== system lib_transmission2/final drive <fd>/model&interface/model/enhancedToWorkspace6 ==
  In1 : Inport
  To Workspace : ToWorkspace  VariableName=fd_trq_out_r  SampleTime=-1
  wires:
  In1/1 -> To Workspace/1

== system lib_transmission2/final drive <fd>/model&interface/model/enhancedToWorkspace7 ==
  In1 : Inport
  To Workspace : ToWorkspace  VariableName=fd_spd_out_r  SampleTime=-1
  wires:
  In1/1 -> To Workspace/1

== system lib_transmission2/final drive <fd>/model&interface/model/help ==

== system lib_transmission2/final drive <fd>/model&interface/model/loss (Nm) ==
  note: The loss torque is zero when the gears are not turning,
      | and is applied at the input side of the gear reduction.
  fd output speed (rad/s) : Inport
  Constant : Constant  Value=0
  Switch : Switch  Threshold=eps  SaturateOnIntegerOverflow=on  InputSameDT=on
  final drive loss torque (Nm) : Constant  Value=fd_loss
  drag torque (Nm) : Outport  InitialOutput=0
  wires:
  final drive loss torque (Nm)/1 -> Switch/1
  Switch/1 -> drag torque (Nm)/1
  fd output speed (rad/s)/1 -> Switch/2
  Constant/1 -> Switch/3

== system lib_transmission2/gearbox <gb>/gearbox model & interface/gearbox model/Block NOTES ==
  note: This gearbox model includes loss data, rotational inertia, and a gear reduction.
  note: The loss torque is zero when the gears are not turning,
      | and is applied at the input side of the gear reduction.
  note: The inertia torque is the input torque required to accelerate the
      | final drive's inertia as measured on the input side.
  note: Available output torque is estimated assuming that the gearbox efficiency for theavailable input
      | torque andspeed is the same as the gearbox efficiency for the REQUESTED input torque.
  note: This is a good assumption, at least for the VW 4-speed manual transaxle of SAE 820741.
      | In the VW transaxle, efficiency is fairly independent of torque and speed at high torques.

== system lib_transmission2/gearbox <gb>/gearbox model & interface/gearbox model/Pout/Pin neglecting inertia ==
  note: Pout/Pin, neglecting inertia, is used to estimate the output torque given the
      | input torque in a very simple forward-facing calculation.
  Tin : Inport
  Tinertia : Inport  Port=2
  Tout : Inport  Port=3
  gear ratio : Inport  Port=4
  Constant1 : Constant  Value=0
  Pout/Pin (neglecting inertia) : Subsystem
      mask Display: disp('/')
  Product : Product  SaturateOnIntegerOverflow=on
  Relational Operator : RelationalOperator  Operator=~=  RndMeth=Nearest  InputSameDT=on
  Saturation : Saturate  UpperLimit=inf  LowerLimit=0
  Switch : Switch  Threshold=eps  SaturateOnIntegerOverflow=on  InputSameDT=on
  Tin-Tinertia : Sum  Inputs=+-  SaturateOnIntegerOverflow=on
  make division bombproof : Subsystem
  Pout/Pin : Outport  InitialOutput=0
  wires:
  Constant1/1 -> Switch/3, Relational Operator/2
  make division bombproof/1(Out1) -> Product/2
  Tinertia/1 -> Tin-Tinertia/2
  Tin/1 -> Tin-Tinertia/1
  Pout/Pin (neglecting inertia)/1(out_1) -> Switch/1
  Relational Operator/1 -> Switch/2
  Switch/1 -> Saturation/1
  Saturation/1 -> Pout/Pin/1
  Tin-Tinertia/1 -> Relational Operator/1, make division bombproof/1(Tin-Tinertia)
  Tout/1 -> Pout/Pin (neglecting inertia)/1(in_1)
  Product/1 -> Pout/Pin (neglecting inertia)/2(in_2)
  gear ratio/1 -> Product/1

== system lib_transmission2/gearbox <gb>/gearbox model & interface/gearbox model/effect of inertia (Nm) ==
  note: The inertia torque is the input torque required to accelerate the
      | gearbox's inertia as measured on the input side.
  gb input speed (rad/s) : Inport
  Gain : Gain  Gain=gb_inertia  SaturateOnIntegerOverflow=on
  d/dt : Derivative
  drag torque (Nm) : Outport  InitialOutput=0
  wires:
  Gain/1 -> drag torque (Nm)/1
  d/dt/1 -> Gain/1
  gb input speed (rad/s)/1 -> d/dt/1

== system lib_transmission2/gearbox <gb>/gearbox model & interface/gearbox model/enhancedToWorkspace ==
  In1 : Inport
  To Workspace : ToWorkspace  VariableName=gb_spd_in_a  SampleTime=-1
  wires:
  In1/1 -> To Workspace/1

== system lib_transmission2/gearbox <gb>/gearbox model & interface/gearbox model/enhancedToWorkspace1 ==
  In1 : Inport
  To Workspace : ToWorkspace  VariableName=gb_trq_in_a  SampleTime=-1
  wires:
  In1/1 -> To Workspace/1

== system lib_transmission2/gearbox <gb>/gearbox model & interface/gearbox model/enhancedToWorkspace2 ==
  In1 : Inport
  To Workspace : ToWorkspace  VariableName=gb_spd_out_a  SampleTime=-1
  wires:
  In1/1 -> To Workspace/1

== system lib_transmission2/gearbox <gb>/gearbox model & interface/gearbox model/enhancedToWorkspace3 ==
  In1 : Inport
  To Workspace : ToWorkspace  VariableName=gb_trq_out_a  SampleTime=-1
  wires:
  In1/1 -> To Workspace/1

== system lib_transmission2/gearbox <gb>/gearbox model & interface/gearbox model/enhancedToWorkspace4 ==
  In1 : Inport
  To Workspace : ToWorkspace  VariableName=gb_ni_trq_out_a  SampleTime=-1
  wires:
  In1/1 -> To Workspace/1

== system lib_transmission2/gearbox <gb>/gearbox model & interface/gearbox model/enhancedToWorkspace5 ==
  In1 : Inport
  To Workspace : ToWorkspace  VariableName=gb_spd_in_r  SampleTime=-1
  wires:
  In1/1 -> To Workspace/1

== system lib_transmission2/gearbox <gb>/gearbox model & interface/gearbox model/enhancedToWorkspace6 ==
  In1 : Inport
  To Workspace : ToWorkspace  VariableName=gb_trq_in_r  SampleTime=-1
  wires:
  In1/1 -> To Workspace/1

== system lib_transmission2/gearbox <gb>/gearbox model & interface/gearbox model/enhancedToWorkspace7 ==
  In1 : Inport
  To Workspace : ToWorkspace  VariableName=gb_spd_out_r  SampleTime=-1
  wires:
  In1/1 -> To Workspace/1

== system lib_transmission2/gearbox <gb>/gearbox model & interface/gearbox model/enhancedToWorkspace8 ==
  In1 : Inport
  To Workspace : ToWorkspace  VariableName=gb_trq_out_r  SampleTime=-1
  wires:
  In1/1 -> To Workspace/1

== system lib_transmission2/gearbox <gb>/gearbox model & interface/gearbox model/enhancedToWorkspace9 ==
  In1 : Inport
  To Workspace : ToWorkspace  VariableName=gb_gear_number  SampleTime=-1
  wires:
  In1/1 -> To Workspace/1
